simulink library "lib_dsphdlmath_v1"  (R2022a)
settings: Solver=ode45  StartTime=0.0  StopTime=10.0  RelTol=1e-3  EnableMultiTasking=on
libraries: simulink x5, lib_dsphdltypes_v1 x3, $bdroot x1
settings Model: Creator=mbabst  LastModifiedBy=mbabst
settings SolverCC: AlgebraicLoopSolver=TrustRegion
settings DataIOCC: LimitDataPoints=on
settings OptimizationCC: LifeSpan=inf
settings DebuggingCC: UnconnectedInputMsg=warning  UnconnectedOutputMsg=warning  UnconnectedLineMsg=warning  AllowSymbolicDim=off  SFUnexpectedBacktrackingDiag=warning  SFNoUnconditionalDefaultTransitionDiag=warning  SFExecutionAtInitializationDiag=none  SFMachineParentedDataDiag=warning  ArithmeticOperatorsInVariantConditions=warning
settings SFSimCC: SimUseLocalCustomCode=off  CustomCodeUndefinedFunction=UseInterfaceOnly
settings RTWCC: RTWUseLocalCustomCode=off  DLArmComputeVersion=19.05
settings CodeAppCC: StateflowObjectComments=on
settings GRTTargetCC: TargetLangStandard=C89/C90 (ANSI)
settings ConfigComp: CovMetricSettings=dw  CovSaveCumulativeToWorkspaceVar=on  CovSaveSingleToWorkspaceVar=on  CovExternalEMLEnable=off

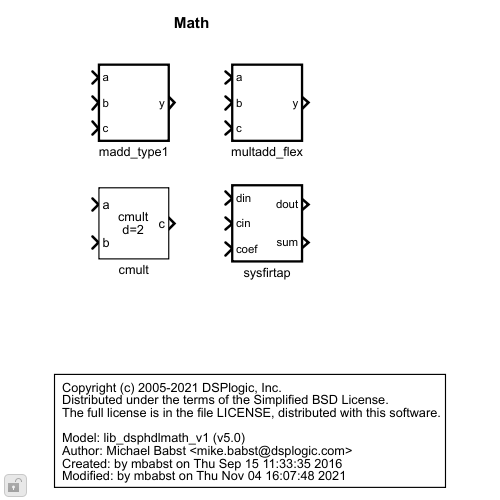
[thumbnail: Simulink's stored preview of the top-level diagram]
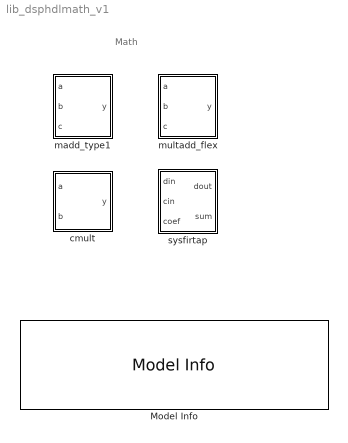
== system lib_dsphdlmath_v1 ==
  note: Math
  Model Info : simulink/Model-Wide Utilities/Model Info  Frame=on  DisplayStringWithTags=|  HorizontalTextAlignment=Left  LeftAlignmentValue=0.02
      | Copyright (c) 2005-2021 DSPlogic, Inc.
      | Distributed under the terms of the Simplified BSD License.
      | The full license is in the file LICENSE, distributed with this software.
      | 
      | Model: %<ModelName> (v%<ModelVersion>)
      | Author: Michael Babst <mike.babst@dsplogic.com>
      | Created: by %<Creator> on %<Created>
      | Modified: by %<ModifiedBy> on %<LastModificationDate>
  cmult : Subsystem  mask(Complex Multiply){Nd_in=1, Nd_out=1}
      mask prompts: Nd_in "Multiplier Input Delay"; Nd_out "Output Delay"
      mask help: Complex multiply operator. This block currently supports only a 4-multiplier implementation.
      mask Display:
      | port_label('output', 1, 'c');
      | port_label('input', 1, 'a')
      | port_label('input', 2, 'b')
      | disp(['cmult\nd=' num2str(Nd_in+Nd_out)])
  madd_type1 : Subsystem  TreatAsAtomicUnit=on  mask(Multiply-Add (Type 1)){Nd_in=1, Nd_out=1, accumMode=Same as C input, addop=++}
      mask prompts: Nd_in "Multiplier Input Delay"; Nd_out "Output Delay"; accumMode "Accumulator Sizing"; addop "Adder Operation"
      mask help:
      | Compute output, y = a*b+c.
      | The a and b inputs and the c output are registered.  The c input is not registered to support lower-latency systolic configurations.
      mask init:
      | madd_type1_init(gcb, accumMode, addop);
      mask TypeOptions accumMode: Automatic | Same as C input
      mask TypeOptions addop: ++ | +- | -+
  multadd_flex : Subsystem  TreatAsAtomicUnit=on  mask(Flexible Multiply-Add){accumMode=Same as C input (after conversion), Nd_in=1, Nd_out=1, Wa=18, extend_a=on, scalingSelect_a=Best Range, Sforce_a=0, roundMode_a=Floor, saturate_a=off, Wb=18, extend_b=on, scalingSelect_b=Best Range, Sforce_b=0, roundMode_b=Floor, saturate_b=off, Wc=63, extend_c=off, scalingSelect_c=Best Range, Sforce_c=60, roundMode_c=Floor, saturate_c=off}
      mask prompts: accumMode "Accumulator sizing"; Nd_in "Multiplier Input Delay"; Nd_out "Output Delay"; Wa "Max width"; extend_a "Extend"; scalingSelect_a "Scaling"; Sforce_a "Scale bits (when forced)"; roundMode_a "Rounding"; saturate_a "Saturate"; Wb "Max width"; extend_b "Extend"; scalingSelect_b "Scaling"; Sforce_b "Scale bits (when forced)"; roundMode_b "Rounding"; saturate_b "Saturate"; Wc "Max width"; extend_c "Extend"; scalingSelect_c "Scaling"; Sforce_c "Scale bits (when forced)"; roundMode_c "Rounding"; saturate_c "Saturate"
      mask help: This multiply-add block adds flexible/automatic input type conversions for targeting distributed logic or DSP slice configurations.
      mask init:
      | multadd_flex_init(gcb,...
      |             accumMode,...
      |             roundMode_a, roundMode_b, roundMode_c, ...
      |             saturate_a,  saturate_b, saturate_c, ...
      |             extend_a, extend_b, extend_c,...
      |             scalingSelect_a, scalingSelect_b, scalingSelect_c...
      | )
      mask TypeOptions accumMode: Automatic | Same as C input (after conversion)
      mask TypeOptions scalingSelect_a: Best Precision | Best Range | Forced
      mask TypeOptions roundMode_a: Floor | Nearest | Convergent
      mask TypeOptions scalingSelect_b: Best Precision | Best Range | Forced
      mask TypeOptions roundMode_b: Floor | Nearest | Convergent
      mask TypeOptions scalingSelect_c: Best Precision | Best Range | Forced
      mask TypeOptions roundMode_c: Floor | Nearest | Convergent
      mask DialogControl Container5 Prompt: Parameters
      mask DialogControl Container3 Prompt: Input Conversion
      mask DialogControl Container26 Prompt: Input A
      mask DialogControl Container26_copy Prompt: Input B
      mask DialogControl Container26_copy_copy Prompt: Input C
  sysfirtap : Subsystem  TreatAsAtomicUnit=on  mask(Systolic FIR Tap){accumMode=Same as C input, addop=++}
      mask prompts: accumMode "Accumulator Sizing"; addop "Adder Operation"
      mask help:
      | Compute output, y = din*coef+c.
      | The din and coef inputs and the y output are registered.
      | The data path offers an additional delayed output that can be used for systolic chains.
      mask init:
      | sysfirtap_init(gcb, accumMode, addop);
      mask TypeOptions accumMode: Automatic | Same as C input
      mask TypeOptions addop: ++ | +- | -+

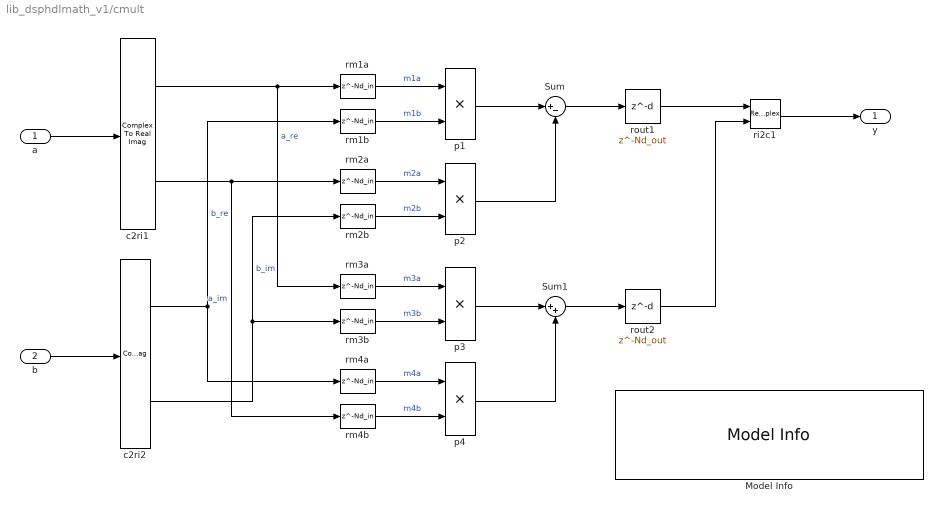
== system lib_dsphdlmath_v1/cmult ==
  a : Inport
  b : Inport  Port=2
  Model Info : simulink/Model-Wide Utilities/Model Info  Frame=on  DisplayStringWithTags=|  HorizontalTextAlignment=Left  LeftAlignmentValue=0.02
      | Copyright (c) 2005-2021 DSPlogic, Inc.
      | Distributed under the terms of the Simplified BSD License.
      | The full license is in the file LICENSE, distributed with this software.
      | 
      | Model: %<ModelName> (v%<ModelVersion>)
      | Author: Michael Babst <mike.babst@dsplogic.com>
      | Created: by %<Creator> on %<Created>
      | Modified: by %<ModifiedBy> on %<LastModificationDate>
  Sum : Sum  Inputs=|+-
  Sum1 : Sum  Inputs=|++
  c2ri1 : ComplexToRealImag
  c2ri2 : ComplexToRealImag
  p{1..4} (4 alike) : Product
  ri2c1 : RealImagToComplex
  rm1a : Delay  DelayLength=Nd_in  InitialCondition=0
  rm1b : Delay  DelayLength=Nd_in  InitialCondition=0
  rm2a : Delay  DelayLength=Nd_in  InitialCondition=0
  rm2b : Delay  DelayLength=Nd_in  InitialCondition=0
  rm3a : Delay  DelayLength=Nd_in  InitialCondition=0
  rm3b : Delay  DelayLength=Nd_in  InitialCondition=0
  rm4a : Delay  DelayLength=Nd_in  InitialCondition=0
  rm4b : Delay  DelayLength=Nd_in  InitialCondition=0
  rout1 : Delay  DelayLength=Nd_out  InitialCondition=0
  rout2 : Delay  DelayLength=Nd_out  InitialCondition=0
  y : Outport
  wires:
  c2ri1/1 -> rm1a/1, rm3a/1  "a_re"
  c2ri1/2 -> rm2a/1, rm4b/1  "a_im"
  c2ri2/1 -> rm4a/1, rm1b/1  "b_re"
  c2ri2/2 -> rm3b/1, rm2b/1  "b_im"
  a/1 -> c2ri1/1
  b/1 -> c2ri2/1
  p1/1 -> Sum/1
  p2/1 -> Sum/2
  p3/1 -> Sum1/1
  p4/1 -> Sum1/2
  Sum/1 -> rout1/1
  Sum1/1 -> rout2/1
  ri2c1/1 -> y/1
  rout1/1 -> ri2c1/1
  rout2/1 -> ri2c1/2
  rm1a/1 -> p1/1  "m1a"
  rm1b/1 -> p1/2  "m1b"
  rm2a/1 -> p2/1  "m2a"
  rm2b/1 -> p2/2  "m2b"
  rm3a/1 -> p3/1  "m3a"
  rm3b/1 -> p3/2  "m3b"
  rm4a/1 -> p4/1  "m4a"
  rm4b/1 -> p4/2  "m4b"

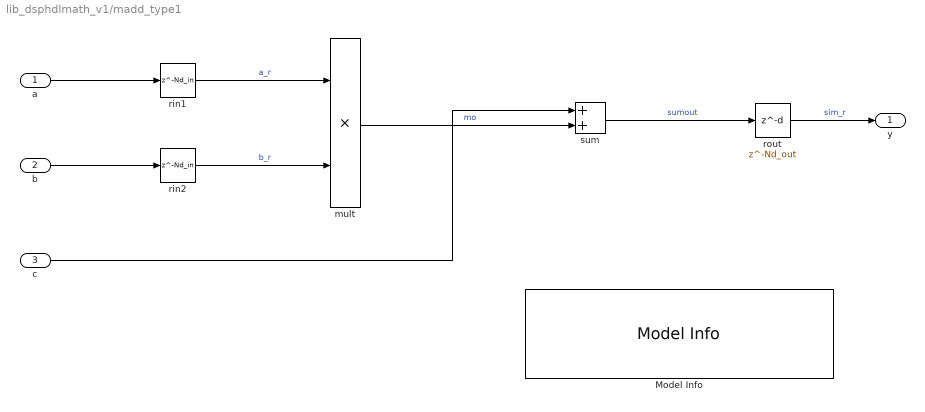
== system lib_dsphdlmath_v1/madd_type1 ==
  a : Inport
  b : Inport  Port=2
  c : Inport  Port=3
  Model Info : simulink/Model-Wide Utilities/Model Info  Frame=on  DisplayStringWithTags=|  HorizontalTextAlignment=Left  LeftAlignmentValue=0.02
      | Copyright (c) 2005-2021 DSPlogic, Inc.
      | Distributed under the terms of the Simplified BSD License.
      | The full license is in the file LICENSE, distributed with this software.
      | 
      | Model: %<ModelName> (v%<ModelVersion>)
      | Author: Michael Babst <mike.babst@dsplogic.com>
      | Created: by %<Creator> on %<Created>
      | Modified: by %<ModifiedBy> on %<LastModificationDate>
  mult : Product
  rin1 : Delay  DelayLength=Nd_in  InitialCondition=0
  rin2 : Delay  DelayLength=Nd_in  InitialCondition=0
  rout : Delay  DelayLength=Nd_out  InitialCondition=0
  sum : Sum  OutDataTypeStr=Inherit: Same as accumulator
      settings: AttributesFormatString=%<AccumDataTypeStr>
  y : Outport
  wires:
  c/1 -> sum/1
  rin1/1 -> mult/1  "a_r"
  rin2/1 -> mult/2  "b_r"
  sum/1 -> rout/1  "sumout"
  rout/1 -> y/1  "sim_r"
  a/1 -> rin1/1
  b/1 -> rin2/1
  mult/1 -> sum/2  "mo"

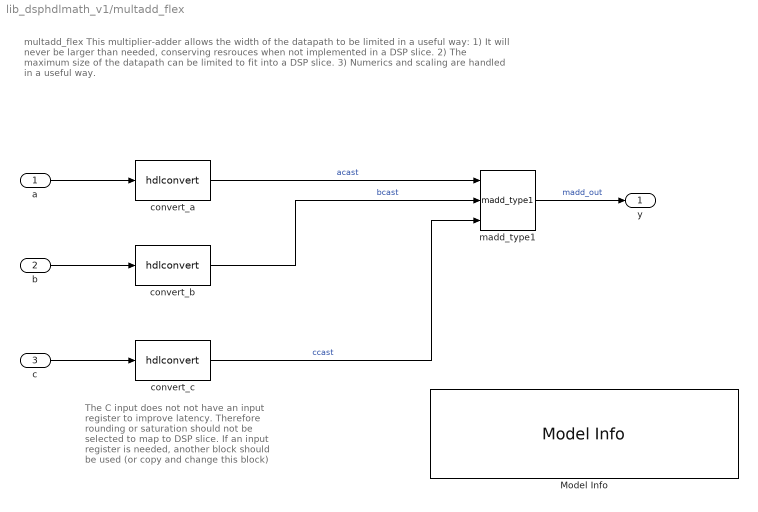
== system lib_dsphdlmath_v1/multadd_flex ==
  note: The C input does not not have an input register to improve latency. Therefore rounding or saturation should not be selected to map to DSP slice. If an input register is needed, another block should be used (or copy and change this block)
  note: multadd_flex
      | This multiplier-adder allows the width of the datapath to be limited in a useful way:
      | 1) It will never be larger than needed, conserving resrouces when not implemented in a DSP slice.
      | 2) The maximum size of the datapath can be limited to fit into a DSP slice.
      | 3) Numerics and scaling are handled in a useful way.
  a : Inport
  b : Inport  Port=2
  c : Inport  Port=3
  Model Info : simulink/Model-Wide Utilities/Model Info  Frame=on  DisplayStringWithTags=|  HorizontalTextAlignment=Left  LeftAlignmentValue=0.02
      | Copyright (c) 2005-2021 DSPlogic, Inc.
      | Distributed under the terms of the Simplified BSD License.
      | The full license is in the file LICENSE, distributed with this software.
      | 
      | Model: %<ModelName> (v%<ModelVersion>)
      | Author: Michael Babst <mike.babst@dsplogic.com>
      | Created: by %<Creator> on %<Created>
      | Modified: by %<ModifiedBy> on %<LastModificationDate>
  convert_a : lib_dsphdltypes_v1/hdlconvert  signed=Inherit  maxwidth=Wa  extend=on  scaleopt=Best Range  Sforce=0  roundMode=Floor  saturate=off
      settings: SourceProductName=DSPHDL Library
  convert_b : lib_dsphdltypes_v1/hdlconvert  signed=Inherit  maxwidth=Wb  extend=on  scaleopt=Best Range  Sforce=0  roundMode=Floor  saturate=off
      settings: SourceProductName=DSPHDL Library
  convert_c : lib_dsphdltypes_v1/hdlconvert  signed=Inherit  maxwidth=Wc  extend=off  scaleopt=Best Range  Sforce=60  roundMode=Floor  saturate=off
      settings: SourceProductName=DSPHDL Library
  madd_type1 : $bdroot/madd_type1  Nd_in=Nd_in  Nd_out=Nd_out  addop=++
  y : Outport
  wires:
  a/1 -> convert_a/1
  b/1 -> convert_b/1
  madd_type1/1 -> y/1  "madd_out"
  c/1 -> convert_c/1
  convert_a/1 -> madd_type1/1  "acast"
  convert_b/1 -> madd_type1/2  "bcast"
  convert_c/1 -> madd_type1/3  "ccast"

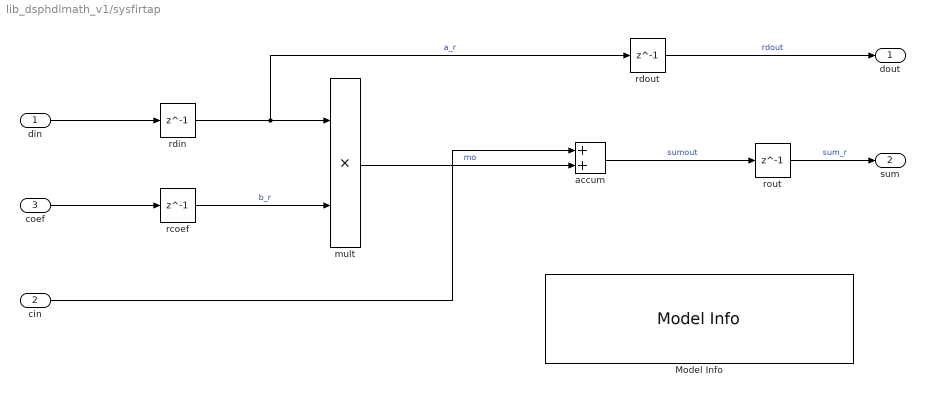
== system lib_dsphdlmath_v1/sysfirtap ==
  din : Inport
  cin : Inport  Port=2
  coef : Inport  Port=3
  Model Info : simulink/Model-Wide Utilities/Model Info  Frame=on  DisplayStringWithTags=|  HorizontalTextAlignment=Left  LeftAlignmentValue=0.02
      | Copyright (c) 2005-2021 DSPlogic, Inc.
      | Distributed under the terms of the Simplified BSD License.
      | The full license is in the file LICENSE, distributed with this software.
      | 
      | Model: %<ModelName> (v%<ModelVersion>)
      | Author: Michael Babst <mike.babst@dsplogic.com>
      | Created: by %<Creator> on %<Created>
      | Modified: by %<ModifiedBy> on %<LastModificationDate>
  accum : Sum  OutDataTypeStr=Inherit: Same as accumulator
      settings: AttributesFormatString=%<AccumDataTypeStr>
  mult : Product
  rcoef : Delay  DelayLength=1  InitialCondition=0
  rdin : Delay  DelayLength=1  InitialCondition=0
  rdout : Delay  DelayLength=1  InitialCondition=0
  rout : Delay  DelayLength=1  InitialCondition=0
  dout : Outport
  sum : Outport  Port=2
  wires:
  cin/1 -> accum/1
  rdin/1 -> rdout/1, mult/1  "a_r"
  rcoef/1 -> mult/2  "b_r"
  accum/1 -> rout/1  "sumout"
  rout/1 -> sum/1  "sum_r"
  din/1 -> rdin/1
  coef/1 -> rcoef/1
  mult/1 -> accum/2  "mo"
  rdout/1 -> dout/1  "rdout"
